simulink model "gm_sampleModel2037_sub"  (R2023a)
settings: Solver=VariableStepAuto  StartTime=0.0  StopTime=10.0  RelTol=1e-3
libraries: hdlsllib x1
settings Model: Creator=user1  LastModifiedBy=user1
settings OptimizationCC: BlockReduction=off  ConditionallyExecuteInputs=off
settings DebuggingCC: InheritedTsInSrcMsg=none

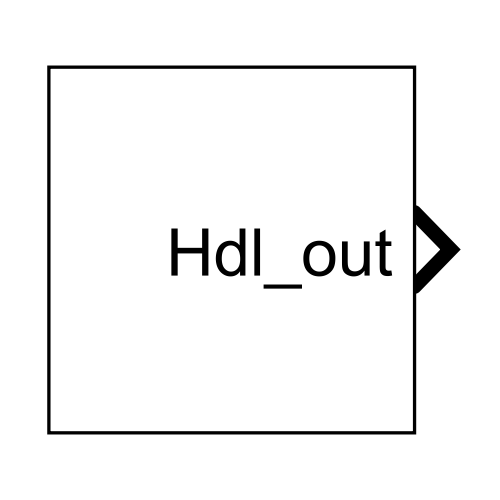
[thumbnail: Simulink's stored preview of the top-level diagram]
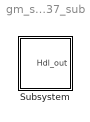
== system gm_sampleModel2037_sub ==
  Subsystem : Subsystem

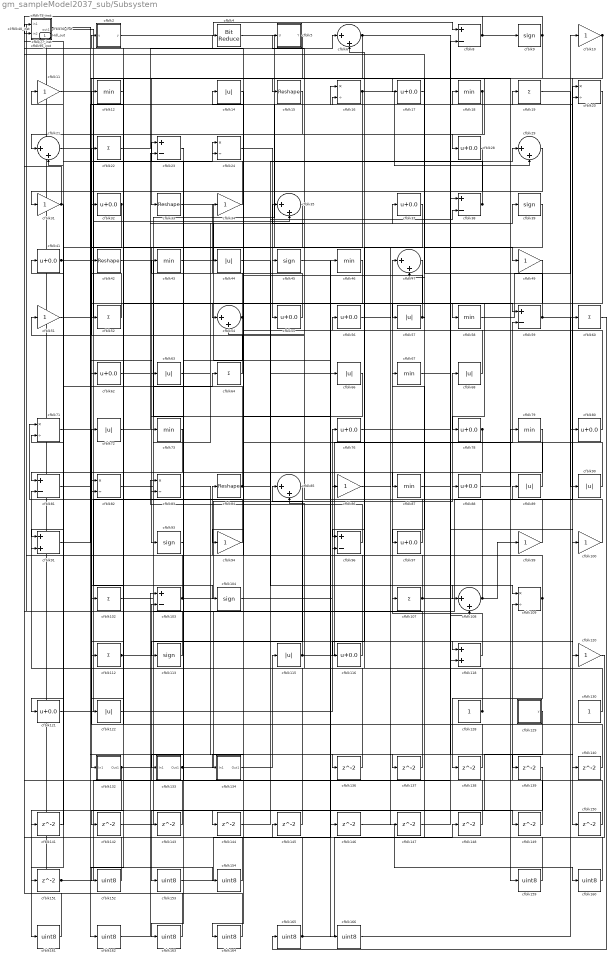
== system gm_sampleModel2037_sub/Subsystem ==
  cfblk{10..11,31,34,49,51,86,94,99..100,120} (11 alike) : Gain  OutDataTypeStr=uint8
  cfblk{19,22,52,60,64,102,107,112} (8 alike) : Sum  Inputs=+  OutDataTypeStr=uint8
  cfblk{8,23,38,59,81,96,103} (7 alike) : Sum  Inputs=+-  OutDataTypeStr=uint8
  cfblk{9,39,45,93,104,113} (6 alike) : Signum
  cfblk105_inst : Subsystem
  cfblk{6,21,29,35,47,54,85,108} (8 alike) : Sum  Inputs=|++  OutDataTypeStr=uint8
  cfblk{16,20,24,71,82..83,109} (7 alike) : Product  Inputs=*/  OutDataTypeStr=uint8  RndMeth=Zero  SaturateOnIntegerOverflow=on
  cfblk110_inst : Subsystem
  cfblk{14,44,57,63,66,68,72,89..90,115,122} (11 alike) : Abs  OutDataTypeStr=uint8  SaturateOnIntegerOverflow=off
  cfblk{17,28,32,37,41,55..56,62,76,78,80,88,97,116,121} (15 alike) : Bias  Bias=0.0  SaturateOnIntegerOverflow=off
  cfblk118 : Sum  OutDataTypeStr=uint8
  cfblk{12,18,43,46,58,67,73,79,87} (9 alike) : MinMax  OutDataTypeStr=uint8
  cfblk128 : Constant  OutDataTypeStr=uint8  SampleTime=-1
  cfblk129 : Subsystem  mask(Counter Limited){uplimit=double(7), tsamp=double(-1)}
      mask prompts: uplimit "Simulink:masks:UpperLimit_MP"; tsamp "Simulink:masks:SampleTime_MP"
      mask help: Simulink:masks:CounterLimited_MD
      mask init:
      | nbits = double(8);
      | tsamp = double(-1);
      | uplimit = double(7);
  cfblk130 : Constant  OutDataTypeStr=uint8  SampleTime=-1
  cfblk132 : Subsystem
  cfblk133 : Subsystem
  cfblk134 : Subsystem
  cfblk{136..151} (16 alike) : Delay  SampleTime=1
  cfblk13_inst : Subsystem
  cfblk{15,33,42,84} (4 alike) : Reshape
  cfblk{152..154,159..166} (11 alike) : DataTypeConversion  OutDataTypeStr=uint8  SaturateOnIntegerOverflow=off  RndMeth=Floor
  cfblk2 : Subsystem  mask(Compare To Constant){relop=<=, const=double(3), OutDataTypeStr=uint8, ZeroCross=on}
      mask prompts: relop "Simulink:masks:Operator_MP"; const "Simulink:masks:ConstantValue_MP"; OutDataTypeStr "Simulink:masks:OutputDataType_MP"; ZeroCross "Simulink:masks:EnableZerocrossingDetection_MP"
      mask help: Simulink:masks:CompareToConstant_MD
      mask init:
      | OutDataTypeStr = 'uint8';
      | ZeroCross = 'on';
      | blkName = 'sampleModel2037_sub/Subsystem/cfblk2';
      | const = double(3);
      | const_str = '3.0';
      | const_val = double(3);
      | relop = '<=';
      | setValue = 'fixdt(0, 8)';
      | str = '<= 3';
      mask TypeOptions relop: == | ~= | < | <= | >= | >
      mask TypeOptions OutDataTypeStr: Simulink:masks:uint8 | Simulink:masks:boolean
      mask Callback ZeroCross: sl('zeroCrossEnable', gcbh);
      mask Display: disp(str)
  cfblk25_inst : Subsystem
  cfblk3 : Constant  Value=0  OutDataTypeStr=uint8  SampleTime=1
  cfblk30_inst : Subsystem
  cfblk4 : hdlsllib/Logic and Bit Operations/Bit Reduce  mode=AND
  cfblk40_inst : Subsystem
  cfblk5 : Subsystem  mask(Detect Rise Nonnegative){vinit=double(0), InputProcessing=Elements as channels (sample based), OutDataTypeStr=uint8}
      mask prompts: vinit "Simulink:masks:InitialCondition_MP"; InputProcessing "Simulink:masks:InputProcessing_MP"; OutDataTypeStr "Simulink:masks:OutputDataType_MP"
      mask help: Simulink:masks:DetectRiseNonnegative_MD
      mask init:
      | InputProcessing = 'Elements as channels (sample based)';
      | OutDataTypeStr = 'uint8';
      | vinit = double(0);
      mask TypeOptions InputProcessing: Simulink:masks:ColumnsAsChannelsFrameBased | Simulink:masks:ElementsAsChannelsSampleBased
      mask TypeOptions OutDataTypeStr: Simulink:masks:uint8 | Simulink:masks:boolean
      mask Display: fprintf('U >= 0\n&  NOT\nU/z >= 0')
  cfblk75_inst : Subsystem
  cfblk77_inst : Subsystem
  cfblk91 : Sum  OutDataTypeStr=uint8
  cfblk95_inst : Subsystem
  Hdl_out : Outport  OutDataTypeStr=uint8  SampleTime=1
  wires:
  cfblk10/1 -> cfblk33/1, cfblk150/1, cfblk132/1(In1)
  cfblk100/1 -> cfblk68/1
  cfblk102/1 -> cfblk64/1
  cfblk103/1 -> cfblk88/1, cfblk81/2
  cfblk104/1 -> cfblk76/1
  cfblk105_inst/1(out1) -> cfblk104/1
  cfblk107/1 -> cfblk89/1, cfblk84/1
  cfblk108/1 -> cfblk54/2, cfblk99/1
  cfblk109/1 -> cfblk75_inst/1(in1), cfblk72/1, cfblk138/1
  cfblk11/1 -> cfblk49/1
  cfblk110_inst/1(out1) -> cfblk58/1
  cfblk112/1 -> cfblk118/1, cfblk12/1
  cfblk113/1 -> cfblk75_inst/2(in2)
  cfblk115/1 -> cfblk85/1, cfblk59/2
  cfblk116/1 -> cfblk24/1
  cfblk118/1 -> cfblk47/1
  cfblk12/1 -> cfblk82/1
  cfblk120/1 -> cfblk145/1
  cfblk121/1 -> cfblk66/1
  cfblk122/1 -> cfblk86/1
  cfblk128/1 -> cfblk85/2, cfblk6/2
  cfblk129/1(y) -> cfblk153/1
  cfblk13_inst/1(out1) -> cfblk159/1
  cfblk130/1 -> cfblk41/1
  cfblk132/1(Out1) -> cfblk161/1, cfblk107/1
  cfblk133/1(Out1) -> cfblk96/2, cfblk20/1
  cfblk134/1(Out1) -> cfblk115/1
  cfblk136/1 -> cfblk71/2
  cfblk137/1 -> cfblk40_inst/2(in2)
  cfblk138/1 -> cfblk82/2
  cfblk139/1 -> cfblk163/1
  cfblk14/1 -> cfblk144/1
  cfblk140/1 -> cfblk2/1(u)
  cfblk141/1 -> cfblk21/2
  cfblk142/1 -> cfblk20/2
  cfblk143/1 -> cfblk110_inst/1(in1)
  cfblk144/1 -> cfblk38/2
  cfblk145/1 -> cfblk91/2
  cfblk146/1 -> cfblk160/1
  cfblk147/1 -> cfblk8/2
  cfblk148/1 -> cfblk23/1
  cfblk149/1 -> cfblk109/2
  cfblk15/1 -> cfblk21/1
  cfblk150/1 -> cfblk103/2
  cfblk151/1 -> cfblk108/2, Hdl_out/1
  cfblk152/1 -> cfblk30_inst/2(in2)
  cfblk153/1 -> cfblk46/1
  cfblk154/1 -> cfblk30_inst/1(in1)
  cfblk159/1 -> cfblk67/1
  cfblk16/1 -> cfblk93/1, cfblk29/2
  cfblk160/1 -> cfblk13_inst/1(in1)
  cfblk161/1 -> cfblk13_inst/2(in2)
  cfblk162/1 -> cfblk103/1
  cfblk163/1 -> cfblk77_inst/1(in1)
  cfblk164/1 -> cfblk77_inst/2(in2)
  cfblk165/1 -> cfblk95_inst/1(in1), cfblk148/1
  cfblk166/1 -> cfblk60/1
  cfblk17/1 -> cfblk57/1
  cfblk18/1 -> cfblk62/1, cfblk118/2
  cfblk19/1 -> cfblk80/1
  cfblk2/1(y) -> cfblk8/1
  cfblk20/1 -> cfblk94/1
  cfblk21/1 -> cfblk24/2
  cfblk22/1 -> cfblk6/1
  cfblk23/1 -> cfblk73/1
  cfblk24/1 -> cfblk55/1
  cfblk25_inst/1(out1) -> cfblk17/1
  cfblk28/1 -> cfblk164/1
  cfblk29/1 -> cfblk143/1
  cfblk3/1 -> cfblk154/1
  cfblk30_inst/1(out1) -> cfblk45/1
  cfblk31/1 -> cfblk121/1, cfblk105_inst/1(in1)
  cfblk32/1 -> cfblk81/1, cfblk151/1
  cfblk33/1 -> cfblk166/1
  cfblk34/1 -> cfblk40_inst/1(in1)
  cfblk35/1 -> cfblk122/1
  cfblk37/1 -> cfblk96/1
  cfblk38/1 -> cfblk110_inst/2(in2), cfblk31/1
  cfblk39/1 -> cfblk87/1
  cfblk4/1 -> cfblk147/1
  cfblk40_inst/1(out1) -> cfblk54/1, cfblk136/1
  cfblk41/1 -> cfblk35/2, cfblk16/2
  cfblk42/1 -> cfblk146/1
  cfblk43/1 -> cfblk39/1
  cfblk44/1 -> cfblk108/1
  cfblk45/1 -> cfblk120/1
  cfblk46/1 -> cfblk152/1
  cfblk47/1 -> cfblk116/1
  cfblk49/1 -> cfblk78/1
  cfblk5/1(Y) -> cfblk102/1
  cfblk51/1 -> cfblk16/1
  cfblk52/1 -> cfblk22/1
  cfblk54/1 -> cfblk83/2, cfblk43/1
  cfblk55/1 -> cfblk34/1
  cfblk56/1 -> cfblk140/1
  cfblk57/1 -> cfblk97/1, cfblk4/1
  cfblk58/1 -> cfblk10/1
  cfblk59/1 -> cfblk90/1, cfblk105_inst/2(in2)
  cfblk6/1 -> cfblk59/1, cfblk15/1
  cfblk60/1 -> cfblk165/1
  cfblk62/1 -> cfblk23/2
  cfblk63/1 -> cfblk37/1
  cfblk64/1 -> cfblk42/1
  cfblk66/1 -> cfblk134/1(In1)
  cfblk67/1 -> cfblk19/1
  cfblk68/1 -> cfblk35/1
  cfblk71/1 -> cfblk32/1
  cfblk72/1 -> cfblk38/1
  cfblk73/1 -> cfblk91/1
  cfblk75_inst/1(out1) -> cfblk63/1
  cfblk76/1 -> cfblk139/1
  cfblk77_inst/1(out1) -> cfblk162/1
  cfblk78/1 -> cfblk142/1, cfblk141/1
  cfblk79/1 -> cfblk112/1
  cfblk8/1 -> cfblk95_inst/2(in2), cfblk9/1
  cfblk80/1 -> cfblk25_inst/1(in1)
  cfblk81/1 -> cfblk18/1
  cfblk82/1 -> cfblk44/1
  cfblk83/1 -> cfblk137/1
  cfblk84/1 -> cfblk29/1, cfblk11/1
  cfblk85/1 -> cfblk113/1
  cfblk86/1 -> cfblk109/1
  cfblk87/1 -> cfblk100/1
  cfblk88/1 -> cfblk79/1
  cfblk89/1 -> cfblk14/1
  cfblk9/1 -> cfblk47/2, cfblk28/1, cfblk25_inst/2(in2)
  cfblk90/1 -> cfblk56/1
  cfblk91/1 -> cfblk52/1
  cfblk93/1 -> cfblk133/1(In1)
  cfblk94/1 -> cfblk71/1
  cfblk95_inst/1(out1) -> cfblk149/1
  cfblk96/1 -> cfblk83/1
  cfblk97/1 -> cfblk5/1(U)
  cfblk99/1 -> cfblk51/1

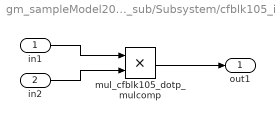
== system gm_sampleModel2037_sub/Subsystem/cfblk105_inst ==
  in1 : Inport  OutDataTypeStr=uint8  SampleTime=1
  in2 : Inport  Port=2  OutDataTypeStr=uint8  SampleTime=1
  mul_cfblk105_dotp_mulcomp : Product  Inputs=**  OutDataTypeStr=uint8  SampleTime=1
  out1 : Outport  OutDataTypeStr=uint8  SampleTime=1
  wires:
  in1/1 -> mul_cfblk105_dotp_mulcomp/1
  in2/1 -> mul_cfblk105_dotp_mulcomp/2
  mul_cfblk105_dotp_mulcomp/1 -> out1/1

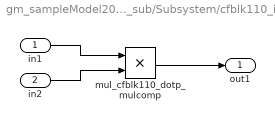
== system gm_sampleModel2037_sub/Subsystem/cfblk110_inst ==
  in1 : Inport  OutDataTypeStr=uint8  SampleTime=1
  in2 : Inport  Port=2  OutDataTypeStr=uint8  SampleTime=1
  mul_cfblk110_dotp_mulcomp : Product  Inputs=**  OutDataTypeStr=uint8  SampleTime=1
  out1 : Outport  OutDataTypeStr=uint8  SampleTime=1
  wires:
  in1/1 -> mul_cfblk110_dotp_mulcomp/1
  in2/1 -> mul_cfblk110_dotp_mulcomp/2
  mul_cfblk110_dotp_mulcomp/1 -> out1/1

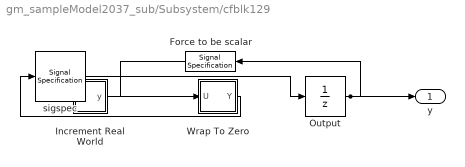
== system gm_sampleModel2037_sub/Subsystem/cfblk129 ==
  Force to be scalar : SignalSpecification  DisableCoverage=on  Dimensions=1
  Increment Real World : Subsystem  mask(Real World Value Increment){}
      mask help: Simulink:masks:RealWorldValueIncrement_MD
      mask Display: disp('V++')
  Output : UnitDelay  InitialCondition=0.0  SampleTime=tsamp  HasFrameUpgradeWarning=on
  Wrap To Zero : Subsystem  mask(Wrap To Zero){Threshold=double(7)}
      mask prompts: Threshold "Simulink:masks:Threshold_MP"
      mask help: Simulink:masks:WrapToZero_MD
  sigspec : SignalSpecification  OutDataTypeStr=uint8  Dimensions=1
  y : Outport  SampleTime=1
  wires:
  Force to be scalar/1 -> Increment Real World/1(u)
  Increment Real World/1(y) -> Wrap To Zero/1(U)
  Output/1 -> Force to be scalar/1, y/1
  Wrap To Zero/1(Y) -> sigspec/1
  sigspec/1 -> Output/1

== system gm_sampleModel2037_sub/Subsystem/cfblk132 ==
  In1 : Inport  OutDataTypeStr=uint8  PortDimensions=1  SampleTime=1
  Out1 : Outport  SampleTime=1
  wires:
  In1/1 -> Out1/1

== system gm_sampleModel2037_sub/Subsystem/cfblk133 ==
  In1 : Inport  OutDataTypeStr=uint8  PortDimensions=1  SampleTime=1
  Out1 : Outport  SampleTime=1
  wires:
  In1/1 -> Out1/1

== system gm_sampleModel2037_sub/Subsystem/cfblk134 ==
  In1 : Inport  OutDataTypeStr=uint8  PortDimensions=1  SampleTime=1
  Out1 : Outport  SampleTime=1
  wires:
  In1/1 -> Out1/1

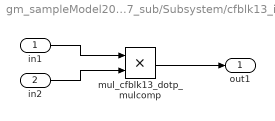
== system gm_sampleModel2037_sub/Subsystem/cfblk13_inst ==
  in1 : Inport  OutDataTypeStr=uint8  SampleTime=1
  in2 : Inport  Port=2  OutDataTypeStr=uint8  SampleTime=1
  mul_cfblk13_dotp_mulcomp : Product  Inputs=**  OutDataTypeStr=uint8  SampleTime=1
  out1 : Outport  OutDataTypeStr=uint8  SampleTime=1
  wires:
  in1/1 -> mul_cfblk13_dotp_mulcomp/1
  in2/1 -> mul_cfblk13_dotp_mulcomp/2
  mul_cfblk13_dotp_mulcomp/1 -> out1/1

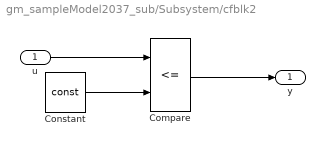
== system gm_sampleModel2037_sub/Subsystem/cfblk2 ==
  u : Inport  OutDataTypeStr=uint8  SampleTime=1
  Compare : RelationalOperator  Operator=<=  OutDataTypeStr=fixdt(0, 8)
  Constant : Constant  DisableCoverage=on  Value=const  OutDataTypeStr=Inherit: Inherit via back propagation  SampleTime=-1
  y : Outport  SampleTime=1
  wires:
  u/1 -> Compare/1
  Compare/1 -> y/1
  Constant/1 -> Compare/2

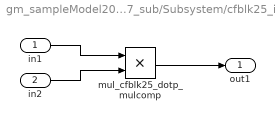
== system gm_sampleModel2037_sub/Subsystem/cfblk25_inst ==
  in1 : Inport  OutDataTypeStr=uint8  SampleTime=1
  in2 : Inport  Port=2  OutDataTypeStr=uint8  SampleTime=1
  mul_cfblk25_dotp_mulcomp : Product  Inputs=**  OutDataTypeStr=uint8  SampleTime=1
  out1 : Outport  OutDataTypeStr=uint8  SampleTime=1
  wires:
  in1/1 -> mul_cfblk25_dotp_mulcomp/1
  in2/1 -> mul_cfblk25_dotp_mulcomp/2
  mul_cfblk25_dotp_mulcomp/1 -> out1/1

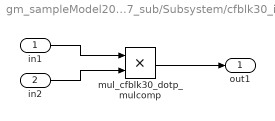
== system gm_sampleModel2037_sub/Subsystem/cfblk30_inst ==
  in1 : Inport  OutDataTypeStr=uint8  SampleTime=1
  in2 : Inport  Port=2  OutDataTypeStr=uint8  SampleTime=1
  mul_cfblk30_dotp_mulcomp : Product  Inputs=**  OutDataTypeStr=uint8  SampleTime=1
  out1 : Outport  OutDataTypeStr=uint8  SampleTime=1
  wires:
  in1/1 -> mul_cfblk30_dotp_mulcomp/1
  in2/1 -> mul_cfblk30_dotp_mulcomp/2
  mul_cfblk30_dotp_mulcomp/1 -> out1/1

== system gm_sampleModel2037_sub/Subsystem/cfblk40_inst ==
  in1 : Inport  OutDataTypeStr=uint8  SampleTime=1
  in2 : Inport  Port=2  OutDataTypeStr=uint8  SampleTime=1
  mul_cfblk40_dotp_mulcomp : Product  Inputs=**  OutDataTypeStr=uint8  SampleTime=1
  out1 : Outport  OutDataTypeStr=uint8  SampleTime=1
  wires:
  in1/1 -> mul_cfblk40_dotp_mulcomp/1
  in2/1 -> mul_cfblk40_dotp_mulcomp/2
  mul_cfblk40_dotp_mulcomp/1 -> out1/1

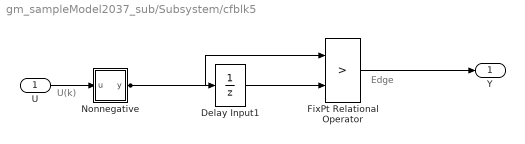
== system gm_sampleModel2037_sub/Subsystem/cfblk5 ==
  note: U(k)
  note: Edge
  U : Inport  OutDataTypeStr=uint8  SampleTime=1
  Delay Input1 : UnitDelay  Description=Store in Global RAM  DisableCoverage=on  InitialCondition=vinit  SampleTime=-1  HasFrameUpgradeWarning=on
  FixPt Relational Operator : RelationalOperator  Operator=>  OutDataTypeStr=fixdt(0, 8)  ZeroCross=off  InputSameDT=off
  Nonnegative : Subsystem  mask(Compare To Zero){relop=>=, OutDataTypeStr=boolean, ZeroCross=off}
      mask prompts: relop "Simulink:masks:Operator_MP"; OutDataTypeStr "Simulink:masks:OutputDataType_MP"; ZeroCross "Simulink:masks:EnableZerocrossingDetection_MP"
      mask help: Simulink:masks:CompareToZero_MD
      mask init:
      | OutDataTypeStr = 'boolean';
      | ZeroCross = 'off';
      | blkName = 'sampleModel2037_sub/Subsystem/cfblk5/Nonnegative';
      | relop = '>=';
      | setValue = 'boolean';
      mask TypeOptions relop: == | ~= | < | <= | >= | >
      mask TypeOptions OutDataTypeStr: Simulink:masks:uint8 | Simulink:masks:boolean
      mask Callback ZeroCross: sl('zeroCrossEnable', gcbh);
      mask Display: disp([relop,' 0'])
  Y : Outport  SampleTime=1
  wires:
  U/1 -> Nonnegative/1(u)
  Delay Input1/1 -> FixPt Relational Operator/2
  FixPt Relational Operator/1 -> Y/1
  Nonnegative/1(y) -> FixPt Relational Operator/1, Delay Input1/1

== system gm_sampleModel2037_sub/Subsystem/cfblk75_inst ==
  in1 : Inport  OutDataTypeStr=uint8  SampleTime=1
  in2 : Inport  Port=2  OutDataTypeStr=uint8  SampleTime=1
  mul_cfblk75_dotp_mulcomp : Product  Inputs=**  OutDataTypeStr=uint8  SampleTime=1
  out1 : Outport  OutDataTypeStr=uint8  SampleTime=1
  wires:
  in1/1 -> mul_cfblk75_dotp_mulcomp/1
  in2/1 -> mul_cfblk75_dotp_mulcomp/2
  mul_cfblk75_dotp_mulcomp/1 -> out1/1

== system gm_sampleModel2037_sub/Subsystem/cfblk77_inst ==
  in1 : Inport  OutDataTypeStr=uint8  SampleTime=1
  in2 : Inport  Port=2  OutDataTypeStr=uint8  SampleTime=1
  mul_cfblk77_dotp_mulcomp : Product  Inputs=**  OutDataTypeStr=uint8  SampleTime=1
  out1 : Outport  OutDataTypeStr=uint8  SampleTime=1
  wires:
  in1/1 -> mul_cfblk77_dotp_mulcomp/1
  in2/1 -> mul_cfblk77_dotp_mulcomp/2
  mul_cfblk77_dotp_mulcomp/1 -> out1/1

== system gm_sampleModel2037_sub/Subsystem/cfblk95_inst ==
  in1 : Inport  OutDataTypeStr=uint8  SampleTime=1
  in2 : Inport  Port=2  OutDataTypeStr=uint8  SampleTime=1
  mul_cfblk95_dotp_mulcomp : Product  Inputs=**  OutDataTypeStr=uint8  SampleTime=1
  out1 : Outport  OutDataTypeStr=uint8  SampleTime=1
  wires:
  in1/1 -> mul_cfblk95_dotp_mulcomp/1
  in2/1 -> mul_cfblk95_dotp_mulcomp/2
  mul_cfblk95_dotp_mulcomp/1 -> out1/1

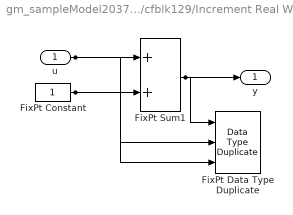
== system gm_sampleModel2037_sub/Subsystem/cfblk129/Increment Real World ==
  u : Inport  OutDataTypeStr=uint8  SampleTime=1
  FixPt Constant : Constant  DisableCoverage=on  OutDataTypeStr=Inherit: Inherit via back propagation  SampleTime=-1
  FixPt Data Type Duplicate : DataTypeDuplicate  DisableCoverage=on  NumInputPorts=3
  FixPt Sum1 : Sum  InputSameDT=on  OutDataTypeStr=Inherit: Inherit via back propagation  LockScale=on
  y : Outport  SampleTime=1
  wires:
  u/1 -> FixPt Sum1/1, FixPt Data Type Duplicate/2
  FixPt Constant/1 -> FixPt Sum1/2, FixPt Data Type Duplicate/3
  FixPt Sum1/1 -> FixPt Data Type Duplicate/1, y/1

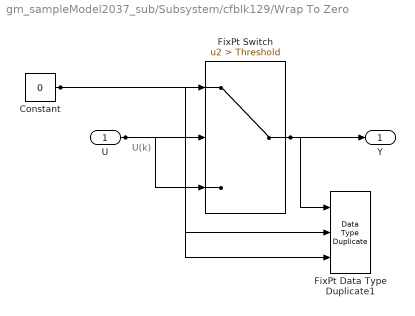
== system gm_sampleModel2037_sub/Subsystem/cfblk129/Wrap To Zero ==
  note: U(k)
  U : Inport  OutDataTypeStr=uint8  SampleTime=1
  Constant : Constant  DisableCoverage=on  Value=0  OutDataTypeStr=Inherit: Inherit via back propagation  SampleTime=-1
  FixPt Data Type Duplicate1 : DataTypeDuplicate  DisableCoverage=on  NumInputPorts=3
  FixPt Switch : Switch  Criteria=u2 > Threshold  Threshold=Threshold  OutDataTypeStr=Inherit: Inherit via back propagation  ZeroCross=off  SaturateOnIntegerOverflow=off  InputSameDT=off
  Y : Outport  SampleTime=1
  wires:
  U/1 -> FixPt Switch/3, FixPt Switch/2, FixPt Data Type Duplicate1/2
  Constant/1 -> FixPt Switch/1, FixPt Data Type Duplicate1/3
  FixPt Switch/1 -> FixPt Data Type Duplicate1/1, Y/1

== system gm_sampleModel2037_sub/Subsystem/cfblk5/Nonnegative ==
  u : Inport  OutDataTypeStr=uint8  SampleTime=1
  Compare : RelationalOperator  OutDataTypeStr=boolean  ZeroCross=off
  Constant : Constant  DisableCoverage=on  Value=0  OutDataTypeStr=Inherit: Inherit via back propagation  SampleTime=-1  PreserveConstantTs=on
  y : Outport  SampleTime=1
  wires:
  u/1 -> Compare/1
  Compare/1 -> y/1
  Constant/1 -> Compare/2
